simulink model "axis_controller"  (R2014a)
settings: Solver=ode3  StartTime=0.0  StopTime=10.0  FixedStep=0.001  RelTol=1e-3
values from neighbouring files (symbols this model uses):
  v_max = 0.25e3    (= 250)    [cartesian_control_parameters.m]
settings Model: Creator=andy  LastModifiedBy=andy
settings RTWCC: ProcessScript=grt_make_rtw_hook

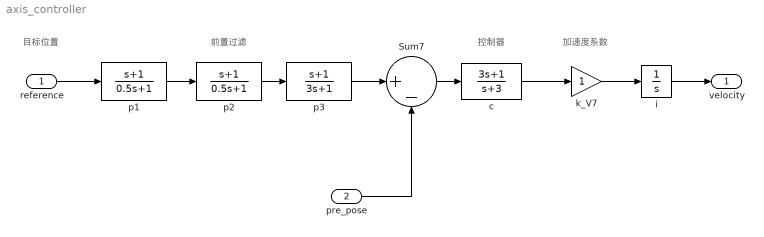
== system axis_controller ==
  note: 加速度系数
  note: 控制器
  note: 前置过滤
  note: 目标位置
  reference : Inport
  pre_pose : Inport  Port=2
  Sum7 : Sum  Inputs=|+-
  c : TransferFcn  Numerator=[3 1]  Denominator=[1 3]
  i : Integrator  LimitOutput=on  UpperSaturationLimit=v_max  LowerSaturationLimit=-v_max
  k_V7 : Gain
  p1 : TransferFcn  Numerator=[1, 1]  Denominator=[0.5 1]
  p2 : TransferFcn  Numerator=[1, 1]  Denominator=[0.5 1]
  "p3 " : TransferFcn  Numerator=[1, 1]  Denominator=[3 1]
  velocity : Outport
  wires:
  c/1 -> k_V7/1
  pre_pose/1 -> Sum7/2
  Sum7/1 -> c/1
  "p3 "/1 -> Sum7/1
  k_V7/1 -> i/1
  i/1 -> velocity/1
  reference/1 -> p1/1
  p2/1 -> "p3 "/1
  p1/1 -> p2/1
